simulink model "CT_models"  (R2019b)
settings: Solver=VariableStepAuto  StartTime=0.0  StopTime=20  RelTol=1e-3
values from neighbouring files (symbols this model uses):
  Atot = [0 1 0 0 0 0 0 0 ... (first row only)    [06_StringVehicles.m]    (also in project_06_StringVehicles_FrancoSavino.m)
  Btot = [Btot,Bdec{i}]    [LMI_CT_DeDicont.m]    (also in di_fixed_modes.m = [Btot,Baggr{i}]; project_06_StringVehicles_FrancoSavino.m = [[0 1 0 0 0 0 0 0]', [0 0 0 1 0 0 0 0]', [0 0 0 0 0 1 0 0]',)
  Ctot = eye(8)    [06_StringVehicles.m]    (also in di_fixed_modes.m = [Ctot; project_06_StringVehicles_FrancoSavino.m)
  h_c = 0.01    [project_06_StringVehicles_FrancoSavino.m]
  L = double(L)    [LMI_CT_DeDicont.m]    (also in LMI_DT_DeDicont.m)
  xref = [0 0 0 0 0 0 0 0]'    [project_06_StringVehicles_FrancoSavino.m]
undefined symbols (not defined in the file or in its folder): F, G, H, K_Centr_CT, K_Centr_DT, K_CycleBidir_CT, K_CycleBidir_DT, K_CycleUnidir_CT, K_CycleUnidir_DT, K_Decentr_CT, K_Decentr_DT, K_Dist_Star_Bi_CT, K_Dist_Star_Bi_DT, K_Dist_Star_Uni_CT, K_Dist_Star_Uni_DT, K_Inv_CycleUnidir_CT, K_Inv_CycleUnidir_DT
libraries: cstblocks x14
settings Model: Creator=alexm  LastModifiedBy=matte
settings SFSimCC: CustomCodeUndefinedFunction=UseInterfaceOnly

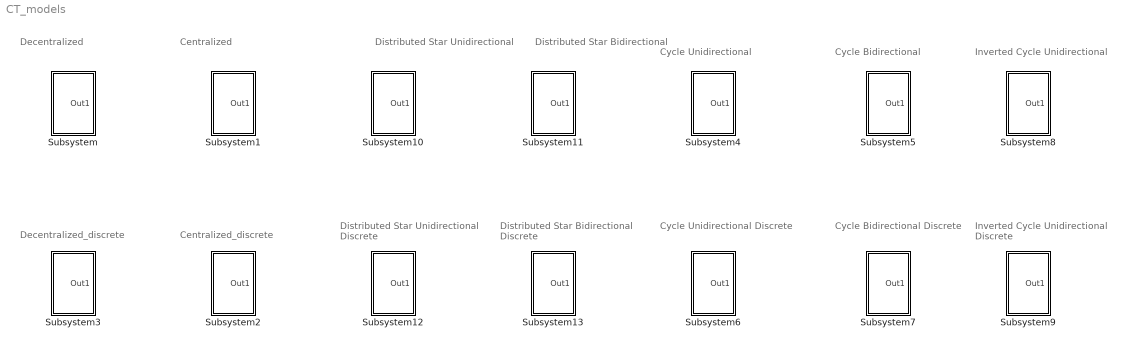
== system CT_models ==
  note: Decentralized
  note: Centralized
  note: Centralized_discrete
  note: Decentralized_discrete
  note: Cycle Unidirectional
  note: Cycle Bidirectional
  note: Cycle Unidirectional Discrete
  note: Cycle Bidirectional Discrete
  note: Inverted Cycle Unidirectional
  note: Inverted Cycle Unidirectional Discrete
  note: Distributed Star Unidirectional
  note: Distributed Star Bidirectional
  note: Distributed Star Unidirectional Discrete
  note: Distributed Star Bidirectional Discrete
  Subsystem : Subsystem
  Subsystem1 : Subsystem
  Subsystem10 : Subsystem
  Subsystem11 : Subsystem
  Subsystem12 : Subsystem
  Subsystem13 : Subsystem
  Subsystem2 : Subsystem
  Subsystem3 : Subsystem
  Subsystem4 : Subsystem
  Subsystem5 : Subsystem
  Subsystem6 : Subsystem
  Subsystem7 : Subsystem
  Subsystem8 : Subsystem
  Subsystem9 : Subsystem

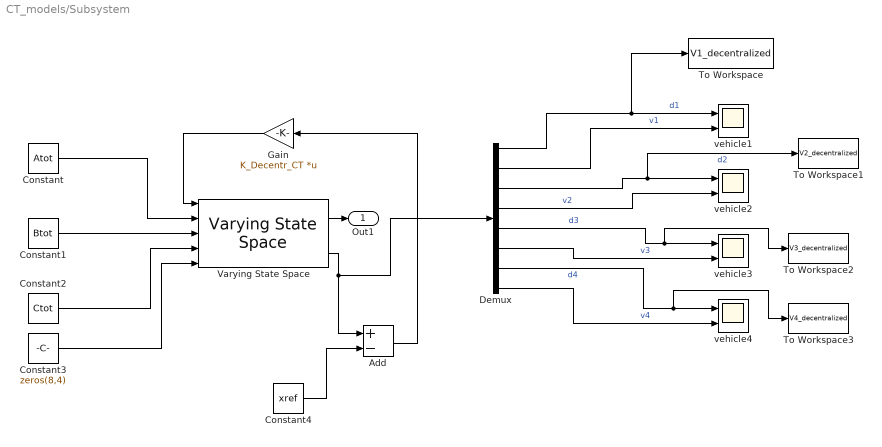
== system CT_models/Subsystem ==
  Add : Sum  Inputs=+-
  Constant : Constant  Value=Atot
  Constant1 : Constant  Value=Btot
  Constant2 : Constant  Value=Ctot
  Constant3 : Constant  Value=zeros(8,4)
  Constant4 : Constant  Value=xref
  Demux : Demux  Outputs=8
  Gain : Gain  Gain=K_Decentr_CT  Multiplication=Matrix(K*u) (u vector)
  To Workspace : ToWorkspace  VariableName=V1_decentralized  SaveFormat=Timeseries  SampleTime=h_c
      settings: Save2DSignal=2-D array (concatenate along first dimension)
  To Workspace1 : ToWorkspace  VariableName=V2_decentralized  SaveFormat=Timeseries  SampleTime=h_c
      settings: Save2DSignal=2-D array (concatenate along first dimension)
  To Workspace2 : ToWorkspace  VariableName=V3_decentralized  SaveFormat=Timeseries  SampleTime=h_c
      settings: Save2DSignal=2-D array (concatenate along first dimension)
  To Workspace3 : ToWorkspace  VariableName=V4_decentralized  SaveFormat=Timeseries  SampleTime=h_c
      settings: Save2DSignal=2-D array (concatenate along first dimension)
  Varying State Space : cstblocks/Linear Parameter Varying/Varying State Space  x0=x0  xNames=''  OutputX=on  OutputDX=off
      settings: SourceProductName=Control System Toolbox
  "vehicle1 " : Scope  NumInputPorts=2
  "vehicle2 " : Scope  NumInputPorts=2
  "vehicle3 " : Scope  NumInputPorts=2
  "vehicle4 " : Scope  NumInputPorts=2
  Out1 : Outport  VectorParamsAs1DForOutWhenUnconnected=off
  wires:
  Constant3/1 -> Varying State Space/5
  Demux/8 -> "vehicle4 "/2  "v4"
  Demux/7 -> To Workspace3/1, "vehicle4 "/1  "d4"
  Demux/5 -> To Workspace2/1, "vehicle3 "/1  "d3"
  Gain/1 -> Varying State Space/1
  Demux/3 -> To Workspace1/1, "vehicle2 "/1  "d2"
  Demux/1 -> To Workspace/1, "vehicle1 "/1  "d1"
  Demux/6 -> "vehicle3 "/2  "v3"
  Demux/4 -> "vehicle2 "/2  "v2"
  Constant1/1 -> Varying State Space/3
  Constant/1 -> Varying State Space/2
  Varying State Space/1 -> Out1/1
  Demux/2 -> "vehicle1 "/2  "v1"
  Constant2/1 -> Varying State Space/4
  Constant4/1 -> Add/2
  Add/1 -> Gain/1
  Varying State Space/2 -> Add/1, Demux/1

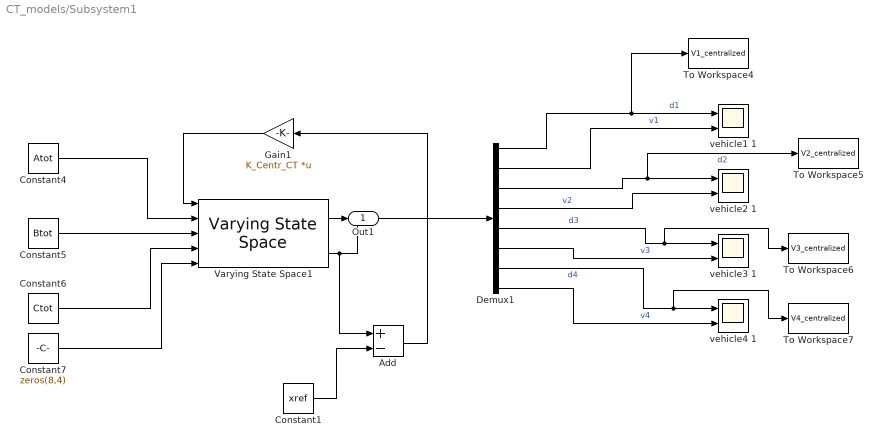
== system CT_models/Subsystem1 ==
  Add : Sum  Inputs=+-
  Constant1 : Constant  Value=xref
  Constant4 : Constant  Value=Atot
  Constant5 : Constant  Value=Btot
  Constant6 : Constant  Value=Ctot
  Constant7 : Constant  Value=zeros(8,4)
  Demux1 : Demux  Outputs=8
  Gain1 : Gain  Gain=K_Centr_CT  Multiplication=Matrix(K*u) (u vector)
  To Workspace4 : ToWorkspace  VariableName=V1_centralized  SaveFormat=Timeseries  SampleTime=h_c
      settings: Save2DSignal=2-D array (concatenate along first dimension)
  To Workspace5 : ToWorkspace  VariableName=V2_centralized  SaveFormat=Timeseries  SampleTime=h_c
      settings: Save2DSignal=2-D array (concatenate along first dimension)
  To Workspace6 : ToWorkspace  VariableName=V3_centralized  SaveFormat=Timeseries  SampleTime=h_c
      settings: Save2DSignal=2-D array (concatenate along first dimension)
  To Workspace7 : ToWorkspace  VariableName=V4_centralized  SaveFormat=Timeseries  SampleTime=h_c
      settings: Save2DSignal=2-D array (concatenate along first dimension)
  Varying State Space1 : cstblocks/Linear Parameter Varying/Varying State Space  x0=x0  xNames=''  OutputX=on  OutputDX=off
      settings: SourceProductName=Control System Toolbox
  vehicle1 1 : Scope  NumInputPorts=2
  vehicle2 1 : Scope  NumInputPorts=2
  vehicle3 1 : Scope  NumInputPorts=2
  vehicle4 1 : Scope  NumInputPorts=2
  Out1 : Outport  VectorParamsAs1DForOutWhenUnconnected=off
  wires:
  Gain1/1 -> Varying State Space1/1
  Demux1/7 -> To Workspace7/1, vehicle4 1/1  "d4"
  Demux1/5 -> To Workspace6/1, vehicle3 1/1  "d3"
  Demux1/1 -> To Workspace4/1, vehicle1 1/1  "d1"
  Constant6/1 -> Varying State Space1/4
  Constant4/1 -> Varying State Space1/2
  Varying State Space1/1 -> Out1/1
  Constant5/1 -> Varying State Space1/3
  Demux1/8 -> vehicle4 1/2  "v4"
  Demux1/6 -> vehicle3 1/2  "v3"
  Demux1/4 -> vehicle2 1/2  "v2"
  Demux1/3 -> To Workspace5/1, vehicle2 1/1  "d2"
  Constant7/1 -> Varying State Space1/5
  Varying State Space1/2 -> Add/1, Demux1/1
  Demux1/2 -> vehicle1 1/2  "v1"
  Constant1/1 -> Add/2
  Add/1 -> Gain1/1

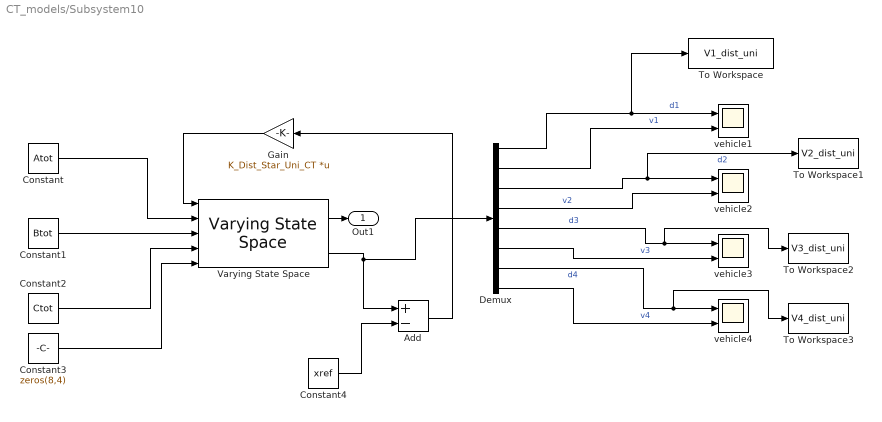
== system CT_models/Subsystem10 ==
  Add : Sum  Inputs=+-
  Constant : Constant  Value=Atot
  Constant1 : Constant  Value=Btot
  Constant2 : Constant  Value=Ctot
  Constant3 : Constant  Value=zeros(8,4)
  Constant4 : Constant  Value=xref
  Demux : Demux  Outputs=8
  Gain : Gain  Gain=K_Dist_Star_Uni_CT  Multiplication=Matrix(K*u) (u vector)
  To Workspace : ToWorkspace  VariableName=V1_dist_uni  SaveFormat=Timeseries  SampleTime=h_c
      settings: Save2DSignal=2-D array (concatenate along first dimension)
  To Workspace1 : ToWorkspace  VariableName=V2_dist_uni  SaveFormat=Timeseries  SampleTime=h_c
      settings: Save2DSignal=2-D array (concatenate along first dimension)
  To Workspace2 : ToWorkspace  VariableName=V3_dist_uni  SaveFormat=Timeseries  SampleTime=h_c
      settings: Save2DSignal=2-D array (concatenate along first dimension)
  To Workspace3 : ToWorkspace  VariableName=V4_dist_uni  SaveFormat=Timeseries  SampleTime=h_c
      settings: Save2DSignal=2-D array (concatenate along first dimension)
  Varying State Space : cstblocks/Linear Parameter Varying/Varying State Space  x0=x0  xNames=''  OutputX=on  OutputDX=off
      settings: SourceProductName=Control System Toolbox
  "vehicle1 " : Scope  NumInputPorts=2
  "vehicle2 " : Scope  NumInputPorts=2
  "vehicle3 " : Scope  NumInputPorts=2
  "vehicle4 " : Scope  NumInputPorts=2
  Out1 : Outport  VectorParamsAs1DForOutWhenUnconnected=off
  wires:
  Constant3/1 -> Varying State Space/5
  Demux/8 -> "vehicle4 "/2  "v4"
  Demux/7 -> To Workspace3/1, "vehicle4 "/1  "d4"
  Demux/5 -> To Workspace2/1, "vehicle3 "/1  "d3"
  Gain/1 -> Varying State Space/1
  Demux/3 -> To Workspace1/1, "vehicle2 "/1  "d2"
  Demux/1 -> To Workspace/1, "vehicle1 "/1  "d1"
  Demux/6 -> "vehicle3 "/2  "v3"
  Demux/4 -> "vehicle2 "/2  "v2"
  Constant1/1 -> Varying State Space/3
  Constant/1 -> Varying State Space/2
  Varying State Space/1 -> Out1/1
  Demux/2 -> "vehicle1 "/2  "v1"
  Constant2/1 -> Varying State Space/4
  Constant4/1 -> Add/2
  Varying State Space/2 -> Demux/1, Add/1
  Add/1 -> Gain/1

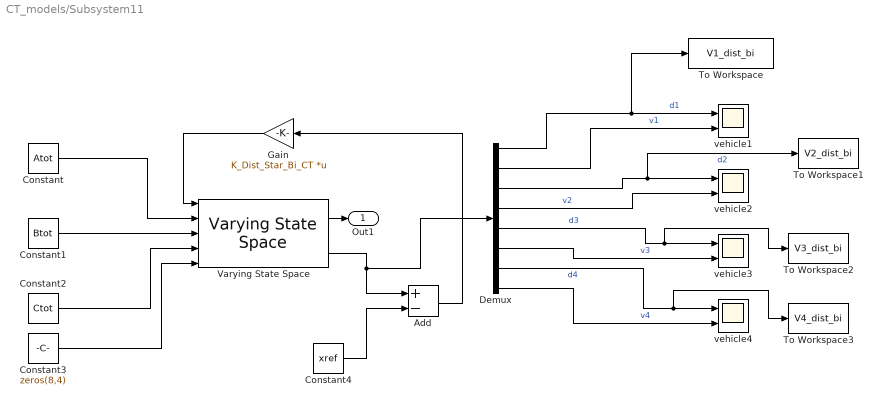
== system CT_models/Subsystem11 ==
  Add : Sum  Inputs=+-
  Constant : Constant  Value=Atot
  Constant1 : Constant  Value=Btot
  Constant2 : Constant  Value=Ctot
  Constant3 : Constant  Value=zeros(8,4)
  Constant4 : Constant  Value=xref
  Demux : Demux  Outputs=8
  Gain : Gain  Gain=K_Dist_Star_Bi_CT  Multiplication=Matrix(K*u) (u vector)
  To Workspace : ToWorkspace  VariableName=V1_dist_bi  SaveFormat=Timeseries  SampleTime=h_c
      settings: Save2DSignal=2-D array (concatenate along first dimension)
  To Workspace1 : ToWorkspace  VariableName=V2_dist_bi  SaveFormat=Timeseries  SampleTime=h_c
      settings: Save2DSignal=2-D array (concatenate along first dimension)
  To Workspace2 : ToWorkspace  VariableName=V3_dist_bi  SaveFormat=Timeseries  SampleTime=h_c
      settings: Save2DSignal=2-D array (concatenate along first dimension)
  To Workspace3 : ToWorkspace  VariableName=V4_dist_bi  SaveFormat=Timeseries  SampleTime=h_c
      settings: Save2DSignal=2-D array (concatenate along first dimension)
  Varying State Space : cstblocks/Linear Parameter Varying/Varying State Space  x0=x0  xNames=''  OutputX=on  OutputDX=off
      settings: SourceProductName=Control System Toolbox
  "vehicle1 " : Scope  NumInputPorts=2
  "vehicle2 " : Scope  NumInputPorts=2
  "vehicle3 " : Scope  NumInputPorts=2
  "vehicle4 " : Scope  NumInputPorts=2
  Out1 : Outport  VectorParamsAs1DForOutWhenUnconnected=off
  wires:
  Constant3/1 -> Varying State Space/5
  Demux/8 -> "vehicle4 "/2  "v4"
  Demux/7 -> To Workspace3/1, "vehicle4 "/1  "d4"
  Demux/5 -> To Workspace2/1, "vehicle3 "/1  "d3"
  Gain/1 -> Varying State Space/1
  Demux/3 -> To Workspace1/1, "vehicle2 "/1  "d2"
  Demux/1 -> To Workspace/1, "vehicle1 "/1  "d1"
  Demux/6 -> "vehicle3 "/2  "v3"
  Demux/4 -> "vehicle2 "/2  "v2"
  Constant1/1 -> Varying State Space/3
  Constant/1 -> Varying State Space/2
  Varying State Space/1 -> Out1/1
  Demux/2 -> "vehicle1 "/2  "v1"
  Constant2/1 -> Varying State Space/4
  Constant4/1 -> Add/2
  Varying State Space/2 -> Demux/1, Add/1
  Add/1 -> Gain/1

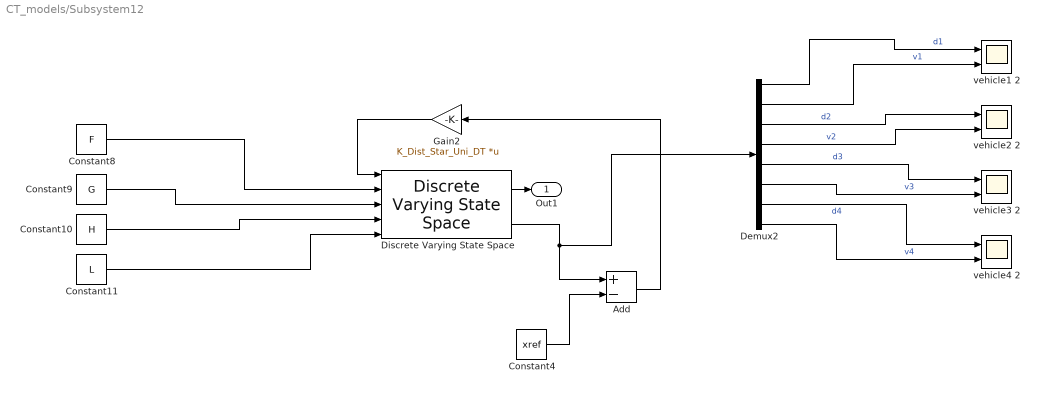
== system CT_models/Subsystem12 ==
  Add : Sum  Inputs=+-
  Constant10 : Constant  Value=H
  Constant11 : Constant  Value=L
  Constant4 : Constant  Value=xref
  Constant8 : Constant  Value=F
  Constant9 : Constant  Value=G
  Demux2 : Demux  Outputs=8
  Discrete Varying State Space : cstblocks/Linear Parameter Varying/Discrete Varying State Space  x0=x0  Ts=0.1  OutputX=on  OutputDX=off
      settings: SourceProductName=Control System Toolbox  SourceProductBaseCode=CT
  Gain2 : Gain  Gain=K_Dist_Star_Uni_DT  Multiplication=Matrix(K*u) (u vector)
  vehicle1 2 : Scope  NumInputPorts=2
  vehicle2 2 : Scope  NumInputPorts=2
  vehicle3 2 : Scope  NumInputPorts=2
  vehicle4 2 : Scope  NumInputPorts=2
  Out1 : Outport  VectorParamsAs1DForOutWhenUnconnected=off
  wires:
  Demux2/2 -> vehicle1 2/2  "v1"
  Constant11/1 -> Discrete Varying State Space/5
  Demux2/7 -> vehicle4 2/1  "d4"
  Demux2/3 -> vehicle2 2/1  "d2"
  Gain2/1 -> Discrete Varying State Space/1
  Demux2/1 -> vehicle1 2/1  "d1"
  Constant9/1 -> Discrete Varying State Space/3
  Constant8/1 -> Discrete Varying State Space/2
  Demux2/5 -> vehicle3 2/1  "d3"
  Demux2/6 -> vehicle3 2/2  "v3"
  Demux2/8 -> vehicle4 2/2  "v4"
  Constant10/1 -> Discrete Varying State Space/4
  Demux2/4 -> vehicle2 2/2  "v2"
  Discrete Varying State Space/1 -> Out1/1
  Constant4/1 -> Add/2
  Discrete Varying State Space/2 -> Demux2/1, Add/1
  Add/1 -> Gain2/1

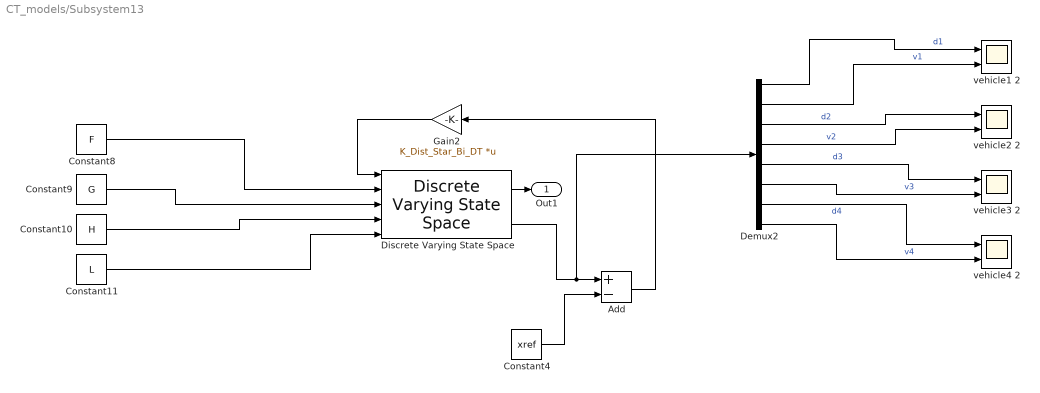
== system CT_models/Subsystem13 ==
  Add : Sum  Inputs=+-
  Constant10 : Constant  Value=H
  Constant11 : Constant  Value=L
  Constant4 : Constant  Value=xref
  Constant8 : Constant  Value=F
  Constant9 : Constant  Value=G
  Demux2 : Demux  Outputs=8
  Discrete Varying State Space : cstblocks/Linear Parameter Varying/Discrete Varying State Space  x0=x0  Ts=0.1  OutputX=on  OutputDX=off
      settings: SourceProductName=Control System Toolbox  SourceProductBaseCode=CT
  Gain2 : Gain  Gain=K_Dist_Star_Bi_DT  Multiplication=Matrix(K*u) (u vector)
  vehicle1 2 : Scope  NumInputPorts=2
  vehicle2 2 : Scope  NumInputPorts=2
  vehicle3 2 : Scope  NumInputPorts=2
  vehicle4 2 : Scope  NumInputPorts=2
  Out1 : Outport  VectorParamsAs1DForOutWhenUnconnected=off
  wires:
  Demux2/2 -> vehicle1 2/2  "v1"
  Constant11/1 -> Discrete Varying State Space/5
  Demux2/7 -> vehicle4 2/1  "d4"
  Demux2/3 -> vehicle2 2/1  "d2"
  Gain2/1 -> Discrete Varying State Space/1
  Demux2/1 -> vehicle1 2/1  "d1"
  Constant9/1 -> Discrete Varying State Space/3
  Constant8/1 -> Discrete Varying State Space/2
  Demux2/5 -> vehicle3 2/1  "d3"
  Demux2/6 -> vehicle3 2/2  "v3"
  Demux2/8 -> vehicle4 2/2  "v4"
  Constant10/1 -> Discrete Varying State Space/4
  Demux2/4 -> vehicle2 2/2  "v2"
  Discrete Varying State Space/1 -> Out1/1
  Constant4/1 -> Add/2
  Discrete Varying State Space/2 -> Demux2/1, Add/1
  Add/1 -> Gain2/1

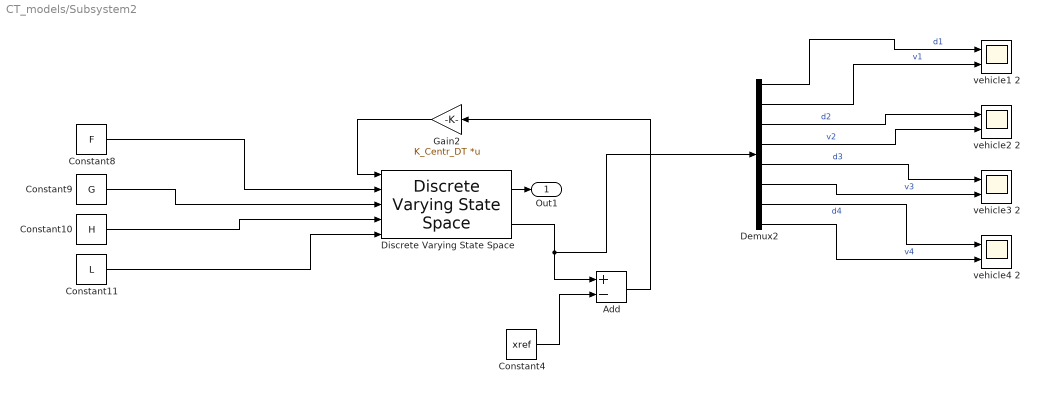
== system CT_models/Subsystem2 ==
  Add : Sum  Inputs=+-
  Constant10 : Constant  Value=H
  Constant11 : Constant  Value=L
  Constant4 : Constant  Value=xref
  Constant8 : Constant  Value=F
  Constant9 : Constant  Value=G
  Demux2 : Demux  Outputs=8
  Discrete Varying State Space : cstblocks/Linear Parameter Varying/Discrete Varying State Space  x0=x0  Ts=0.1  OutputX=on  OutputDX=off
      settings: SourceProductName=Control System Toolbox  SourceProductBaseCode=CT
  Gain2 : Gain  Gain=K_Centr_DT  Multiplication=Matrix(K*u) (u vector)
  vehicle1 2 : Scope  NumInputPorts=2
  vehicle2 2 : Scope  NumInputPorts=2
  vehicle3 2 : Scope  NumInputPorts=2
  vehicle4 2 : Scope  NumInputPorts=2
  Out1 : Outport  VectorParamsAs1DForOutWhenUnconnected=off
  wires:
  Demux2/2 -> vehicle1 2/2  "v1"
  Constant11/1 -> Discrete Varying State Space/5
  Demux2/7 -> vehicle4 2/1  "d4"
  Demux2/3 -> vehicle2 2/1  "d2"
  Gain2/1 -> Discrete Varying State Space/1
  Demux2/1 -> vehicle1 2/1  "d1"
  Constant9/1 -> Discrete Varying State Space/3
  Constant8/1 -> Discrete Varying State Space/2
  Demux2/5 -> vehicle3 2/1  "d3"
  Demux2/6 -> vehicle3 2/2  "v3"
  Demux2/8 -> vehicle4 2/2  "v4"
  Constant10/1 -> Discrete Varying State Space/4
  Demux2/4 -> vehicle2 2/2  "v2"
  Discrete Varying State Space/1 -> Out1/1
  Constant4/1 -> Add/2
  Discrete Varying State Space/2 -> Demux2/1, Add/1
  Add/1 -> Gain2/1

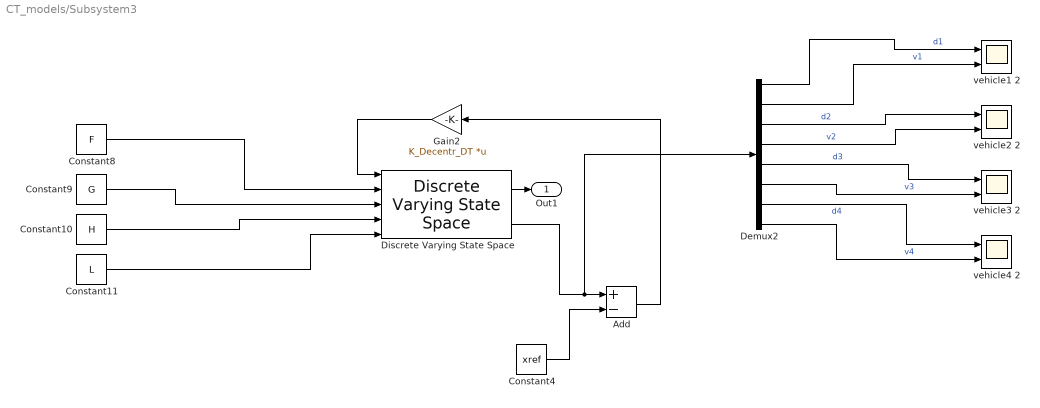
== system CT_models/Subsystem3 ==
  Add : Sum  Inputs=+-
  Constant10 : Constant  Value=H
  Constant11 : Constant  Value=L
  Constant4 : Constant  Value=xref
  Constant8 : Constant  Value=F
  Constant9 : Constant  Value=G
  Demux2 : Demux  Outputs=8
  Discrete Varying State Space : cstblocks/Linear Parameter Varying/Discrete Varying State Space  x0=x0  Ts=0.1  OutputX=on  OutputDX=off
      settings: SourceProductName=Control System Toolbox  SourceProductBaseCode=CT
  Gain2 : Gain  Gain=K_Decentr_DT  Multiplication=Matrix(K*u) (u vector)
  vehicle1 2 : Scope  NumInputPorts=2
  vehicle2 2 : Scope  NumInputPorts=2
  vehicle3 2 : Scope  NumInputPorts=2
  vehicle4 2 : Scope  NumInputPorts=2
  Out1 : Outport  VectorParamsAs1DForOutWhenUnconnected=off
  wires:
  Demux2/7 -> vehicle4 2/1  "d4"
  Demux2/4 -> vehicle2 2/2  "v2"
  Demux2/3 -> vehicle2 2/1  "d2"
  Constant8/1 -> Discrete Varying State Space/2
  Demux2/2 -> vehicle1 2/2  "v1"
  Constant11/1 -> Discrete Varying State Space/5
  Constant9/1 -> Discrete Varying State Space/3
  Demux2/6 -> vehicle3 2/2  "v3"
  Gain2/1 -> Discrete Varying State Space/1
  Demux2/1 -> vehicle1 2/1  "d1"
  Constant10/1 -> Discrete Varying State Space/4
  Demux2/5 -> vehicle3 2/1  "d3"
  Demux2/8 -> vehicle4 2/2  "v4"
  Discrete Varying State Space/1 -> Out1/1
  Constant4/1 -> Add/2
  Discrete Varying State Space/2 -> Demux2/1, Add/1
  Add/1 -> Gain2/1

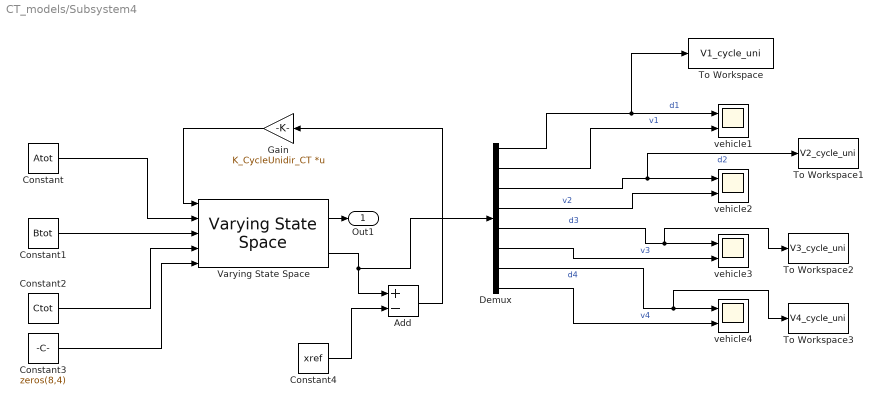
== system CT_models/Subsystem4 ==
  Add : Sum  Inputs=+-
  Constant : Constant  Value=Atot
  Constant1 : Constant  Value=Btot
  Constant2 : Constant  Value=Ctot
  Constant3 : Constant  Value=zeros(8,4)
  Constant4 : Constant  Value=xref
  Demux : Demux  Outputs=8
  Gain : Gain  Gain=K_CycleUnidir_CT  Multiplication=Matrix(K*u) (u vector)
  To Workspace : ToWorkspace  VariableName=V1_cycle_uni  SaveFormat=Timeseries  SampleTime=h_c
      settings: Save2DSignal=2-D array (concatenate along first dimension)
  To Workspace1 : ToWorkspace  VariableName=V2_cycle_uni  SaveFormat=Timeseries  SampleTime=h_c
      settings: Save2DSignal=2-D array (concatenate along first dimension)
  To Workspace2 : ToWorkspace  VariableName=V3_cycle_uni  SaveFormat=Timeseries  SampleTime=h_c
      settings: Save2DSignal=2-D array (concatenate along first dimension)
  To Workspace3 : ToWorkspace  VariableName=V4_cycle_uni  SaveFormat=Timeseries  SampleTime=h_c
      settings: Save2DSignal=2-D array (concatenate along first dimension)
  Varying State Space : cstblocks/Linear Parameter Varying/Varying State Space  x0=x0  xNames=''  OutputX=on  OutputDX=off
      settings: SourceProductName=Control System Toolbox
  "vehicle1 " : Scope  NumInputPorts=2
  "vehicle2 " : Scope  NumInputPorts=2
  "vehicle3 " : Scope  NumInputPorts=2
  "vehicle4 " : Scope  NumInputPorts=2
  Out1 : Outport  VectorParamsAs1DForOutWhenUnconnected=off
  wires:
  Constant3/1 -> Varying State Space/5
  Demux/8 -> "vehicle4 "/2  "v4"
  Demux/7 -> To Workspace3/1, "vehicle4 "/1  "d4"
  Demux/5 -> To Workspace2/1, "vehicle3 "/1  "d3"
  Gain/1 -> Varying State Space/1
  Demux/3 -> To Workspace1/1, "vehicle2 "/1  "d2"
  Demux/1 -> To Workspace/1, "vehicle1 "/1  "d1"
  Demux/6 -> "vehicle3 "/2  "v3"
  Demux/4 -> "vehicle2 "/2  "v2"
  Constant1/1 -> Varying State Space/3
  Constant/1 -> Varying State Space/2
  Varying State Space/1 -> Out1/1
  Demux/2 -> "vehicle1 "/2  "v1"
  Constant2/1 -> Varying State Space/4
  Constant4/1 -> Add/2
  Varying State Space/2 -> Demux/1, Add/1
  Add/1 -> Gain/1

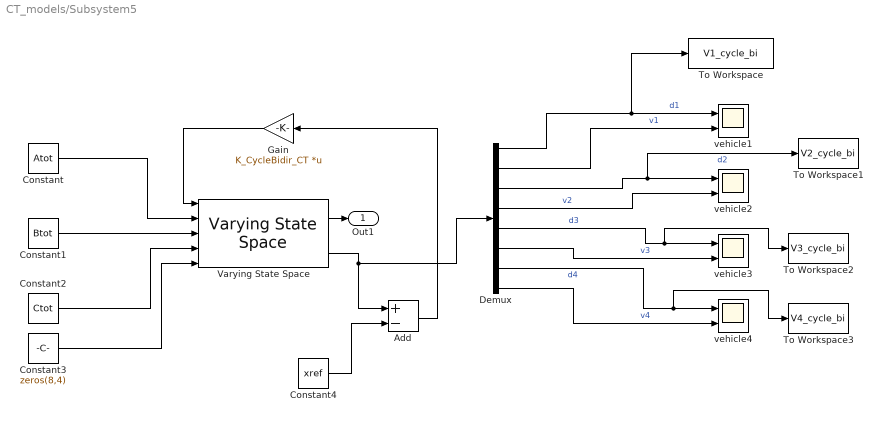
== system CT_models/Subsystem5 ==
  Add : Sum  Inputs=+-
  Constant : Constant  Value=Atot
  Constant1 : Constant  Value=Btot
  Constant2 : Constant  Value=Ctot
  Constant3 : Constant  Value=zeros(8,4)
  Constant4 : Constant  Value=xref
  Demux : Demux  Outputs=8
  Gain : Gain  Gain=K_CycleBidir_CT  Multiplication=Matrix(K*u) (u vector)
  To Workspace : ToWorkspace  VariableName=V1_cycle_bi  SaveFormat=Timeseries  SampleTime=h_c
      settings: Save2DSignal=2-D array (concatenate along first dimension)
  To Workspace1 : ToWorkspace  VariableName=V2_cycle_bi  SaveFormat=Timeseries  SampleTime=h_c
      settings: Save2DSignal=2-D array (concatenate along first dimension)
  To Workspace2 : ToWorkspace  VariableName=V3_cycle_bi  SaveFormat=Timeseries  SampleTime=h_c
      settings: Save2DSignal=2-D array (concatenate along first dimension)
  To Workspace3 : ToWorkspace  VariableName=V4_cycle_bi  SaveFormat=Timeseries  SampleTime=h_c
      settings: Save2DSignal=2-D array (concatenate along first dimension)
  Varying State Space : cstblocks/Linear Parameter Varying/Varying State Space  x0=x0  xNames=''  OutputX=on  OutputDX=off
      settings: SourceProductName=Control System Toolbox
  "vehicle1 " : Scope  NumInputPorts=2
  "vehicle2 " : Scope  NumInputPorts=2
  "vehicle3 " : Scope  NumInputPorts=2
  "vehicle4 " : Scope  NumInputPorts=2
  Out1 : Outport  VectorParamsAs1DForOutWhenUnconnected=off
  wires:
  Constant3/1 -> Varying State Space/5
  Demux/8 -> "vehicle4 "/2  "v4"
  Demux/7 -> To Workspace3/1, "vehicle4 "/1  "d4"
  Demux/5 -> To Workspace2/1, "vehicle3 "/1  "d3"
  Gain/1 -> Varying State Space/1
  Demux/3 -> To Workspace1/1, "vehicle2 "/1  "d2"
  Demux/1 -> To Workspace/1, "vehicle1 "/1  "d1"
  Demux/6 -> "vehicle3 "/2  "v3"
  Demux/4 -> "vehicle2 "/2  "v2"
  Constant1/1 -> Varying State Space/3
  Constant/1 -> Varying State Space/2
  Varying State Space/1 -> Out1/1
  Demux/2 -> "vehicle1 "/2  "v1"
  Constant2/1 -> Varying State Space/4
  Constant4/1 -> Add/2
  Varying State Space/2 -> Add/1, Demux/1
  Add/1 -> Gain/1

== system CT_models/Subsystem6 ==
  Add : Sum  Inputs=+-
  Constant10 : Constant  Value=H
  Constant11 : Constant  Value=L
  Constant4 : Constant  Value=xref
  Constant8 : Constant  Value=F
  Constant9 : Constant  Value=G
  Demux2 : Demux  Outputs=8
  Discrete Varying State Space : cstblocks/Linear Parameter Varying/Discrete Varying State Space  x0=x0  Ts=0.1  OutputX=on  OutputDX=off
      settings: SourceProductName=Control System Toolbox  SourceProductBaseCode=CT
  Gain2 : Gain  Gain=K_CycleUnidir_DT  Multiplication=Matrix(K*u) (u vector)
  vehicle1 2 : Scope  NumInputPorts=2
  vehicle2 2 : Scope  NumInputPorts=2
  vehicle3 2 : Scope  NumInputPorts=2
  vehicle4 2 : Scope  NumInputPorts=2
  Out1 : Outport  VectorParamsAs1DForOutWhenUnconnected=off
  wires:
  Demux2/2 -> vehicle1 2/2  "v1"
  Constant11/1 -> Discrete Varying State Space/5
  Demux2/7 -> vehicle4 2/1  "d4"
  Demux2/3 -> vehicle2 2/1  "d2"
  Gain2/1 -> Discrete Varying State Space/1
  Demux2/1 -> vehicle1 2/1  "d1"
  Constant9/1 -> Discrete Varying State Space/3
  Constant8/1 -> Discrete Varying State Space/2
  Demux2/5 -> vehicle3 2/1  "d3"
  Demux2/6 -> vehicle3 2/2  "v3"
  Demux2/8 -> vehicle4 2/2  "v4"
  Constant10/1 -> Discrete Varying State Space/4
  Demux2/4 -> vehicle2 2/2  "v2"
  Discrete Varying State Space/1 -> Out1/1
  Constant4/1 -> Add/2
  Discrete Varying State Space/2 -> Demux2/1, Add/1
  Add/1 -> Gain2/1

== system CT_models/Subsystem7 ==
  Add : Sum  Inputs=+-
  Constant10 : Constant  Value=H
  Constant11 : Constant  Value=L
  Constant4 : Constant  Value=xref
  Constant8 : Constant  Value=F
  Constant9 : Constant  Value=G
  Demux2 : Demux  Outputs=8
  Discrete Varying State Space : cstblocks/Linear Parameter Varying/Discrete Varying State Space  x0=x0  Ts=0.1  OutputX=on  OutputDX=off
      settings: SourceProductName=Control System Toolbox  SourceProductBaseCode=CT
  Gain2 : Gain  Gain=K_CycleBidir_DT  Multiplication=Matrix(K*u) (u vector)
  vehicle1 2 : Scope  NumInputPorts=2
  vehicle2 2 : Scope  NumInputPorts=2
  vehicle3 2 : Scope  NumInputPorts=2
  vehicle4 2 : Scope  NumInputPorts=2
  Out1 : Outport  VectorParamsAs1DForOutWhenUnconnected=off
  wires:
  Demux2/2 -> vehicle1 2/2  "v1"
  Constant11/1 -> Discrete Varying State Space/5
  Demux2/7 -> vehicle4 2/1  "d4"
  Demux2/3 -> vehicle2 2/1  "d2"
  Gain2/1 -> Discrete Varying State Space/1
  Demux2/1 -> vehicle1 2/1  "d1"
  Constant9/1 -> Discrete Varying State Space/3
  Constant8/1 -> Discrete Varying State Space/2
  Demux2/5 -> vehicle3 2/1  "d3"
  Demux2/6 -> vehicle3 2/2  "v3"
  Demux2/8 -> vehicle4 2/2  "v4"
  Constant10/1 -> Discrete Varying State Space/4
  Demux2/4 -> vehicle2 2/2  "v2"
  Discrete Varying State Space/1 -> Out1/1
  Constant4/1 -> Add/2
  Discrete Varying State Space/2 -> Demux2/1, Add/1
  Add/1 -> Gain2/1

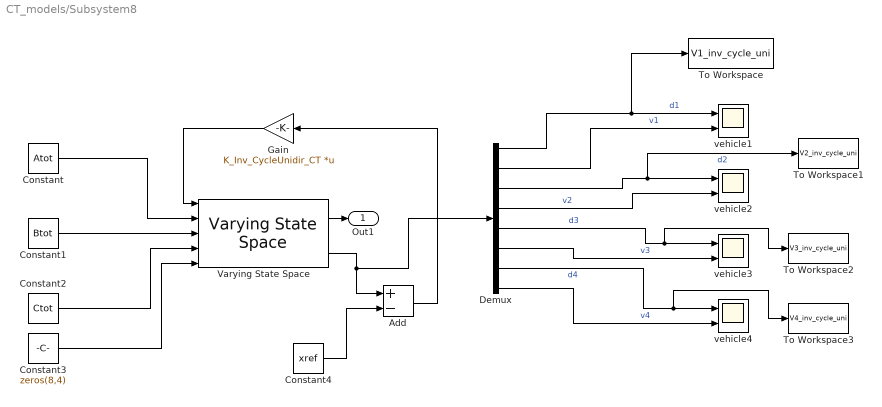
== system CT_models/Subsystem8 ==
  Add : Sum  Inputs=+-
  Constant : Constant  Value=Atot
  Constant1 : Constant  Value=Btot
  Constant2 : Constant  Value=Ctot
  Constant3 : Constant  Value=zeros(8,4)
  Constant4 : Constant  Value=xref
  Demux : Demux  Outputs=8
  Gain : Gain  Gain=K_Inv_CycleUnidir_CT  Multiplication=Matrix(K*u) (u vector)
  To Workspace : ToWorkspace  VariableName=V1_inv_cycle_uni  SaveFormat=Timeseries  SampleTime=h_c
      settings: Save2DSignal=2-D array (concatenate along first dimension)
  To Workspace1 : ToWorkspace  VariableName=V2_inv_cycle_uni  SaveFormat=Timeseries  SampleTime=h_c
      settings: Save2DSignal=2-D array (concatenate along first dimension)
  To Workspace2 : ToWorkspace  VariableName=V3_inv_cycle_uni  SaveFormat=Timeseries  SampleTime=h_c
      settings: Save2DSignal=2-D array (concatenate along first dimension)
  To Workspace3 : ToWorkspace  VariableName=V4_inv_cycle_uni  SaveFormat=Timeseries  SampleTime=h_c
      settings: Save2DSignal=2-D array (concatenate along first dimension)
  Varying State Space : cstblocks/Linear Parameter Varying/Varying State Space  x0=x0  xNames=''  OutputX=on  OutputDX=off
      settings: SourceProductName=Control System Toolbox
  "vehicle1 " : Scope  NumInputPorts=2
  "vehicle2 " : Scope  NumInputPorts=2
  "vehicle3 " : Scope  NumInputPorts=2
  "vehicle4 " : Scope  NumInputPorts=2
  Out1 : Outport  VectorParamsAs1DForOutWhenUnconnected=off
  wires:
  Constant3/1 -> Varying State Space/5
  Demux/8 -> "vehicle4 "/2  "v4"
  Demux/7 -> To Workspace3/1, "vehicle4 "/1  "d4"
  Demux/5 -> To Workspace2/1, "vehicle3 "/1  "d3"
  Gain/1 -> Varying State Space/1
  Demux/3 -> To Workspace1/1, "vehicle2 "/1  "d2"
  Demux/1 -> To Workspace/1, "vehicle1 "/1  "d1"
  Demux/6 -> "vehicle3 "/2  "v3"
  Demux/4 -> "vehicle2 "/2  "v2"
  Constant1/1 -> Varying State Space/3
  Constant/1 -> Varying State Space/2
  Varying State Space/1 -> Out1/1
  Demux/2 -> "vehicle1 "/2  "v1"
  Constant2/1 -> Varying State Space/4
  Constant4/1 -> Add/2
  Varying State Space/2 -> Demux/1, Add/1
  Add/1 -> Gain/1

== system CT_models/Subsystem9 ==
  Add : Sum  Inputs=+-
  Constant10 : Constant  Value=H
  Constant11 : Constant  Value=L
  Constant4 : Constant  Value=xref
  Constant8 : Constant  Value=F
  Constant9 : Constant  Value=G
  Demux2 : Demux  Outputs=8
  Discrete Varying State Space : cstblocks/Linear Parameter Varying/Discrete Varying State Space  x0=x0  Ts=0.1  OutputX=on  OutputDX=off
      settings: SourceProductName=Control System Toolbox  SourceProductBaseCode=CT
  Gain2 : Gain  Gain=K_Inv_CycleUnidir_DT  Multiplication=Matrix(K*u) (u vector)
  vehicle1 2 : Scope  NumInputPorts=2
  vehicle2 2 : Scope  NumInputPorts=2
  vehicle3 2 : Scope  NumInputPorts=2
  vehicle4 2 : Scope  NumInputPorts=2
  Out1 : Outport  VectorParamsAs1DForOutWhenUnconnected=off
  wires:
  Demux2/2 -> vehicle1 2/2  "v1"
  Constant11/1 -> Discrete Varying State Space/5
  Demux2/7 -> vehicle4 2/1  "d4"
  Demux2/3 -> vehicle2 2/1  "d2"
  Gain2/1 -> Discrete Varying State Space/1
  Demux2/1 -> vehicle1 2/1  "d1"
  Constant9/1 -> Discrete Varying State Space/3
  Constant8/1 -> Discrete Varying State Space/2
  Demux2/5 -> vehicle3 2/1  "d3"
  Demux2/6 -> vehicle3 2/2  "v3"
  Demux2/8 -> vehicle4 2/2  "v4"
  Constant10/1 -> Discrete Varying State Space/4
  Demux2/4 -> vehicle2 2/2  "v2"
  Discrete Varying State Space/1 -> Out1/1
  Constant4/1 -> Add/2
  Discrete Varying State Space/2 -> Demux2/1, Add/1
  Add/1 -> Gain2/1
